simulink library "lib1"  (R2016a)
settings: Solver=ode45  StartTime=0.0  StopTime=10.0  RelTol=1e-3
values from neighbouring files (symbols this model uses):
  long_mean_len = short_mean_len * 600    (= 7200)    [rf_controller.m]
  short_mean_len = 12    [rf_controller.m]
settings Model: Creator=jbeau  LastModifiedBy=jbeau
settings DataIOCC: LimitDataPoints=on
settings DebuggingCC: AllowSymbolicDim=off

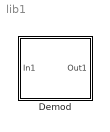
== system lib1 ==
  "Demod " : Subsystem

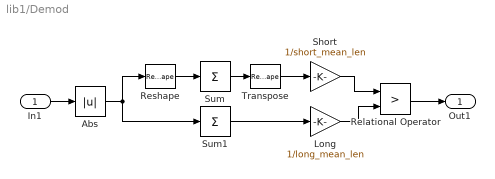
== system lib1/Demod  ==
  In1 : Inport
  Abs : Abs
  Long : Gain  Gain=1/long_mean_len
  Relational Operator : RelationalOperator  Operator=>  OutDataTypeStr=boolean
  Reshape : Reshape  OutputDimensionality=Customize  OutputDimensions=[short_mean_len, 810]
  Short : Gain  Gain=1/short_mean_len
  Sum : Sum  Inputs=+  CollapseMode=Specified dimension
  Sum1 : Sum  Inputs=+  CollapseMode=Specified dimension
  Transpose : Reshape  OutputDimensionality=Column vector (2-D)
  Out1 : Outport
  wires:
  Long/1 -> Relational Operator/2
  Sum1/1 -> Long/1
  Transpose/1 -> Short/1
  Short/1 -> Relational Operator/1
  Abs/1 -> Reshape/1, Sum1/1
  Sum/1 -> Transpose/1
  Reshape/1 -> Sum/1
  In1/1 -> Abs/1
  Relational Operator/1 -> Out1/1
